simulink model "InverterMotorModel"  (R2021a)
settings: Solver=FixedStepAuto  StartTime=0.0  StopTime=t  FixedStep=0.01  RelTol=1e-3
values from neighbouring files (symbols this model uses):
  inv_catastrophic_fault_toggle = input('   0 = no fault  -or-  1 = fault: ')    [Run_GeneratorRectifierBoostConverterInverterMotorModel.m]    (also in Run_InverterMotorModel.m)
  mot_catastrophic_fault_toggle = input('   0 = no fault  -or-  1 = fault: ')    [Run_GeneratorRectifierBoostConverterInverterMotorModel.m]    (also in Run_InverterMotorModel.m)
libraries: PB_Library_Master_Working x2
settings Model: Creator=sfaulk  LastModifiedBy=sfaulk

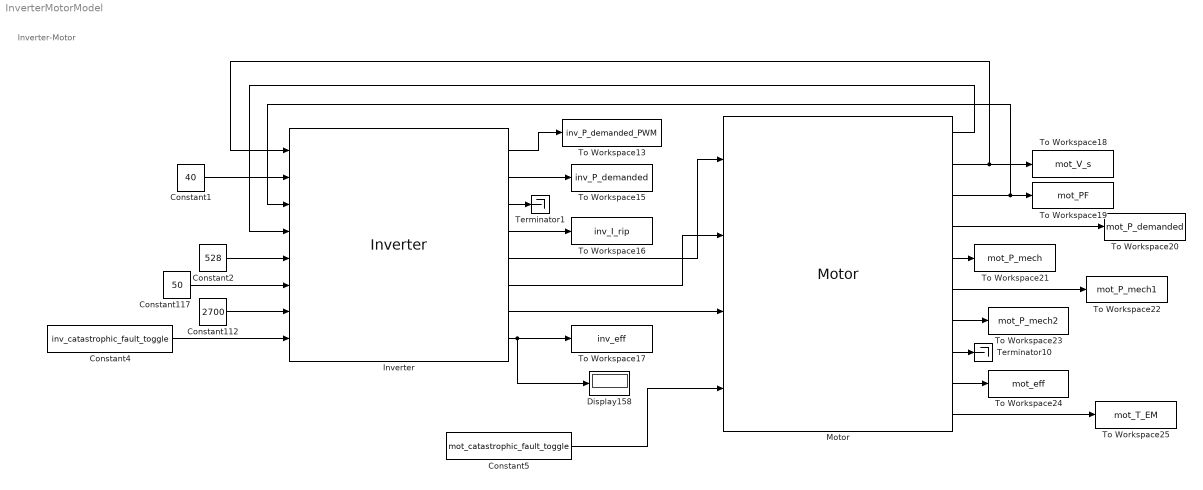
== system InverterMotorModel ==
  note: Inverter-Motor
  Constant1 : Constant  Value=40
  Constant112 : Constant  Value=2700
  Constant117 : Constant  Value=50
  Constant2 : Constant  Value=528
  Constant4 : Constant  Value=inv_catastrophic_fault_toggle
  Constant5 : Constant  Value=mot_catastrophic_fault_toggle
  Display158 : Display
  Inverter : PB_Library_Master_Working/Inverter  T_M=[25 175]  u_D_M=inv_u_D_M  u_ce0_M=[0.971428571428571 0.848275862068965]  R_c_M=[0.0285714285714286 0.0551724137931034]  R_D_M=inv_R_D_M  E0_M=inv_E0_M  E1_M=inv_E1_M  f_sw_M=inv_f_sw_M  L_s_M=0.1  P_max_I=22000  V_phase_I=600  f_sw_I=0  L_s_I=0.1
      link override Goto1: GotoTag=invDF  TagVisibility=global
      link override Goto2: GotoTag=invDI  TagVisibility=global
      link override IGBT Switching Losses/Constant1: Value=0.1
      link override IGBT Switching Losses/Degradation Parameter Multiplier/From14: GotoTag=invDI
      link override IGBT Switching Losses/Degradation Parameter Multiplier/From15: GotoTag=invDF
  Motor : PB_Library_Master_Working/Motor  pp=2.5  flux_m=mot_flux_m  R_s=mot_R_s  L_s=mot_L_s  P_Fe_Nom=mot_P_Fe_Nom  S_nom=mot_S_nom  T_nom=70  P_out_max=22000  I_max=36.5  P_in_max=30000  T_max=80  MassEst_M=-1080970  Poles_i=5  R_s_i=.032  L_s_i=.00086+0.00029  S_nom_i=3000  T_nom_i=70  P_out_max_i=22000  I_max_i=36.5  P_in_max_i=30000  K_i=121  V_nom_i=368  T_max_i=80  CalculatePFe=Compute iron losses automatically  P_Fe_Nom_i=0  I_nom_i=36.5  PF_nom_i=0.99  P_Fe_Calc_Flag=1
      link override Constant8: Value=0.1
      link override Copper Losses/Constant: Value=0.1
      link override Copper Losses/Constant1: Value=0.1
      link override Copper Losses/Degradation Parameter Multiplier/From14: GotoTag=motDI
      link override Copper Losses/Degradation Parameter Multiplier/From15: GotoTag=motDF
      link override Copper Losses/Degradation Parameter Multiplier1/From14: GotoTag=motDI
      link override Copper Losses/Degradation Parameter Multiplier1/From15: GotoTag=motDF
      link override Degradation Parameter Multiplier/From14: GotoTag=motDI
      link override Degradation Parameter Multiplier/From15: GotoTag=motDF
      link override Field Weakening and d current /Constant2: Value=0.1
      link override Field Weakening and d current /Degradation Parameter Multiplier/From14: GotoTag=motDI
      link override Field Weakening and d current /Degradation Parameter Multiplier/From15: GotoTag=motDF
      link override Goto2: TagVisibility=global
      link override Goto3: TagVisibility=global
      link override Iron Loss/Constant1: Value=0.1
      link override Iron Loss/Degradation Parameter Multiplier/From14: GotoTag=motDI
      link override Iron Loss/Degradation Parameter Multiplier/From15: GotoTag=motDF
      link override Vdq/Constant: Value=0.1
      link override Vdq/Constant1: Value=0.1
      link override Vdq/Constant2: Value=0.1
      link override Vdq/Degradation Parameter Multiplier/From14: GotoTag=motDI
      link override Vdq/Degradation Parameter Multiplier/From15: GotoTag=motDF
      link override Vdq/Degradation Parameter Multiplier1/From14: GotoTag=motDI
      link override Vdq/Degradation Parameter Multiplier1/From15: GotoTag=motDF
      link override Vdq/Degradation Parameter Multiplier2/From14: GotoTag=motDI
      link override Vdq/Degradation Parameter Multiplier2/From15: GotoTag=motDF
  Terminator1 : Terminator
  Terminator10 : Terminator
  To Workspace13 : ToWorkspace  VariableName=inv_P_demanded_PWM  SaveFormat=Timeseries  SampleTime=-1
  To Workspace15 : ToWorkspace  VariableName=inv_P_demanded  SaveFormat=Timeseries  SampleTime=-1
  To Workspace16 : ToWorkspace  VariableName=inv_I_rip  SaveFormat=Timeseries  SampleTime=-1
  To Workspace17 : ToWorkspace  VariableName=inv_eff  SaveFormat=Timeseries  SampleTime=-1
  To Workspace18 : ToWorkspace  VariableName=mot_V_s  SaveFormat=Timeseries  SampleTime=-1
  To Workspace19 : ToWorkspace  VariableName=mot_PF  SaveFormat=Timeseries  SampleTime=-1
  To Workspace20 : ToWorkspace  VariableName=mot_P_demanded  SaveFormat=Timeseries  SampleTime=-1
  To Workspace21 : ToWorkspace  VariableName=mot_P_mech  SaveFormat=Timeseries  SampleTime=-1
  To Workspace22 : ToWorkspace  VariableName=mot_P_mech1  SaveFormat=Timeseries  SampleTime=-1
  To Workspace23 : ToWorkspace  VariableName=mot_P_mech2  SaveFormat=Timeseries  SampleTime=-1
  To Workspace24 : ToWorkspace  VariableName=mot_eff  SaveFormat=Timeseries  SampleTime=-1
  To Workspace25 : ToWorkspace  VariableName=mot_T_EM  SaveFormat=Timeseries  SampleTime=-1
  wires:
  Constant2/1 -> Inverter/5
  Inverter/1 -> To Workspace13/1
  Inverter/4 -> To Workspace16/1
  Inverter/6 -> Motor/2
  Motor/8 -> Terminator10/1
  Inverter/5 -> Motor/1
  Inverter/2 -> To Workspace15/1
  Motor/5 -> To Workspace21/1
  Motor/9 -> To Workspace24/1
  Motor/4 -> To Workspace20/1
  Motor/10 -> To Workspace25/1
  Motor/6 -> To Workspace22/1
  Constant5/1 -> Motor/4
  Constant112/1 -> Inverter/7
  Constant117/1 -> Inverter/6
  Inverter/7 -> Motor/3
  Motor/3 -> Inverter/3, To Workspace19/1
  Constant4/1 -> Inverter/8
  Motor/2 -> To Workspace18/1, Inverter/1
  Motor/1 -> Inverter/4
  Inverter/8 -> To Workspace17/1, Display158/1
  Motor/7 -> To Workspace23/1
  Constant1/1 -> Inverter/2
  Inverter/3 -> Terminator1/1
